simulink model "AcermanDynExt"  (R2019b)
settings: Solver=FixedStepAuto  StartTime=0.0  StopTime=simTime  RelTol=1e-3
values from neighbouring files (symbols this model uses):
  a0 = 1    [Ackerman_init.m]
  a1 = 4    [Ackerman_init.m]
  a2 = 3    [Ackerman_init.m]
  Change = 0    [Ackerman_init.m]
  k0 = 1    [Ackerman_init.m]
  k1 = place(Ad,bd,pd)    [Ackerman_init.m]
  k2 = place(Ac,bc,lambdatr')    [Ackerman_init.m]
  l = ylabel('$\omega(t)$' )    [Ackerman_init.m]
  pathType = 1    [Ackerman_init.m]
  phi0 = 0    [Ackerman_init.m]
  r = 2    [Ackerman_init.m]
  ref0 = [0 0]'    [Ackerman_init.m]
  refType = 1    [Ackerman_init.m]
  T = 0.324    [Ackerman_init.m]
  theta0 = pi/2    (= 1.57079632679)    [Ackerman_init.m]
  v0 = 1    [Ackerman_init.m]
  v_ref = 2    [Ackerman_init.m]
  x0 = 1    [Ackerman_init.m]
  y0 = 1    [Ackerman_init.m]
libraries: robotmobilelib x5
(part 1 of 6)
settings Model: Creator=mohd-  LastModifiedBy=mohd-

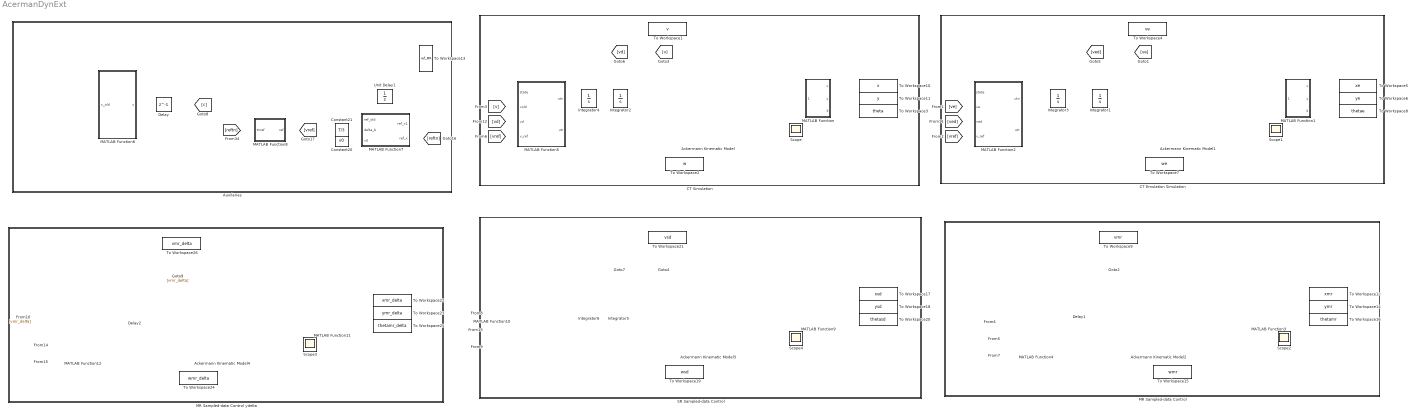
== system AcermanDynExt ==
  Ackermann Kinematic Model{,1..4} (5 alike) : robotmobilelib/Ackermann Kinematic Model  WheelBase=l  VehicleSpeedRange=[-inf inf]  MaxSteeringAngle=pi/3  InitialState=[x0; y0; theta0; phi0]  SimulateUsing=Interpreted execution
      settings: SourceProductName=Robotics System Toolbox  SourceProductBaseCode=RO
  Auxilaries : Subsystem
  CT Emulation Simulation : Subsystem
  CT Simulation : Subsystem
  Constant20 : Constant  Value=v0
  Constant21 : Constant  Value=T/3
  Delay : Delay  DelayLength=1  InitialCondition=0  SampleTime=T/3
  Delay1 : Delay  DelayLength=1  InitialCondition=v0  SampleTime=T
  Delay2 : Delay  DelayLength=1  InitialCondition=v0  SampleTime=T
  Integrator1 : Integrator  InitialCondition=v0
  Integrator2 : Integrator  InitialCondition=v0
  Integrator3 : Integrator
  Integrator4 : Integrator
  Integrator5 : Integrator  InitialCondition=v0
  Integrator6 : Integrator
  MATLAB Function : MATLAB Function  TreatAsAtomicUnit=on
  MATLAB Function1 : MATLAB Function  TreatAsAtomicUnit=on
  MATLAB Function10 : MATLAB Function  TreatAsAtomicUnit=on  SystemSampleTime=T
  MATLAB Function11 : MATLAB Function  TreatAsAtomicUnit=on
  MATLAB Function12 : MATLAB Function  TreatAsAtomicUnit=on  SystemSampleTime=T
  MATLAB Function2 : MATLAB Function  TreatAsAtomicUnit=on  SystemSampleTime=T
  MATLAB Function3 : MATLAB Function  TreatAsAtomicUnit=on
  MATLAB Function4 : MATLAB Function  TreatAsAtomicUnit=on  SystemSampleTime=T
  MATLAB Function5 : MATLAB Function  TreatAsAtomicUnit=on
  MATLAB Function6 : MATLAB Function  TreatAsAtomicUnit=on  SystemSampleTime=T/3
  MATLAB Function7 : MATLAB Function  TreatAsAtomicUnit=on  SystemSampleTime=T
  MATLAB Function8 : MATLAB Function  TreatAsAtomicUnit=on
  MATLAB Function9 : MATLAB Function  TreatAsAtomicUnit=on
  MR Sampled-data Control : Subsystem
  MR Sampled-data Control ydelta : Subsystem
  SR Sampled-data Control : Subsystem
  Scope{,1..4} (5 alike) : Scope
  To Workspace1 : ToWorkspace  VariableName=v  SampleTime=10^-3
      settings: Save2DSignal=2-D array (concatenate along first dimension)
  To Workspace10 : ToWorkspace  VariableName=x  SampleTime=10^-3
      settings: Save2DSignal=2-D array (concatenate along first dimension)
  To Workspace11 : ToWorkspace  VariableName=y  SampleTime=10^-3
      settings: Save2DSignal=2-D array (concatenate along first dimension)
  To Workspace12 : ToWorkspace  VariableName=xmr  SampleTime=10^-3
      settings: Save2DSignal=2-D array (concatenate along first dimension)
  To Workspace13 : ToWorkspace  VariableName=ref_MR  SampleTime=T/3
  To Workspace14 : ToWorkspace  VariableName=ymr  SampleTime=10^-3
      settings: Save2DSignal=2-D array (concatenate along first dimension)
  To Workspace15 : ToWorkspace  VariableName=wmr  SampleTime=10^-3
      settings: Save2DSignal=2-D array (concatenate along first dimension)
  To Workspace16 : ToWorkspace  VariableName=thetamr  SampleTime=10^-3
      settings: Save2DSignal=2-D array (concatenate along first dimension)
  To Workspace17 : ToWorkspace  VariableName=xsd  SampleTime=10^-3
      settings: Save2DSignal=2-D array (concatenate along first dimension)
  To Workspace18 : ToWorkspace  VariableName=ysd  SampleTime=10^-3
      settings: Save2DSignal=2-D array (concatenate along first dimension)
  To Workspace19 : ToWorkspace  VariableName=wsd  SampleTime=10^-3
      settings: Save2DSignal=2-D array (concatenate along first dimension)
  To Workspace2 : ToWorkspace  VariableName=w  SampleTime=10^-3
      settings: Save2DSignal=2-D array (concatenate along first dimension)
  To Workspace20 : ToWorkspace  VariableName=thetasd  SampleTime=10^-3
      settings: Save2DSignal=2-D array (concatenate along first dimension)
  To Workspace21 : ToWorkspace  VariableName=vsd  SampleTime=10^-3
      settings: Save2DSignal=2-D array (concatenate along first dimension)
  To Workspace22 : ToWorkspace  VariableName=xmr_delta  SampleTime=10^-3
      settings: Save2DSignal=2-D array (concatenate along first dimension)
  To Workspace23 : ToWorkspace  VariableName=ymr_delta  SampleTime=10^-3
      settings: Save2DSignal=2-D array (concatenate along first dimension)
  To Workspace24 : ToWorkspace  VariableName=wmr_delta  SampleTime=10^-3
      settings: Save2DSignal=2-D array (concatenate along first dimension)
  To Workspace25 : ToWorkspace  VariableName=thetamr_delta  SampleTime=10^-3
      settings: Save2DSignal=2-D array (concatenate along first dimension)
  To Workspace26 : ToWorkspace  VariableName=vmr_delta  SampleTime=10^-3
      settings: Save2DSignal=2-D array (concatenate along first dimension)
  To Workspace3 : ToWorkspace  VariableName=theta  SampleTime=10^-3
      settings: Save2DSignal=2-D array (concatenate along first dimension)
  To Workspace4 : ToWorkspace  VariableName=ve  SampleTime=10^-3
      settings: Save2DSignal=2-D array (concatenate along first dimension)
  To Workspace5 : ToWorkspace  VariableName=xe  SampleTime=10^-3
      settings: Save2DSignal=2-D array (concatenate along first dimension)
  To Workspace6 : ToWorkspace  VariableName=ye  SampleTime=10^-3
      settings: Save2DSignal=2-D array (concatenate along first dimension)
  To Workspace7 : ToWorkspace  VariableName=we  SampleTime=10^-3
      settings: Save2DSignal=2-D array (concatenate along first dimension)
  To Workspace8 : ToWorkspace  VariableName=thetae  SampleTime=10^-3
      settings: Save2DSignal=2-D array (concatenate along first dimension)
  To Workspace9 : ToWorkspace  VariableName=vmr  SampleTime=10^-3
      settings: Save2DSignal=2-D array (concatenate along first dimension)
  Unit Delay1 : UnitDelay  InitialCondition=ref0  SampleTime=T/3  HasFrameUpgradeWarning=on
  wires:
  Ackermann Kinematic Model3/2 -> Scope4/1
  Ackermann Kinematic Model2/1 -> MATLAB Function4/1(state), MATLAB Function3/1(state)
  [vmr] -> MATLAB Function4/2(v)
  Constant20/1 -> MATLAB Function7/3(v0)
  MATLAB Function9/2(y) -> To Workspace18/1
  Delay1/1 -> To Workspace9/1, [vmr], Ackermann Kinematic Model2/1
  MATLAB Function3/1(x) -> To Workspace12/1
  MATLAB Function3/2(y) -> To Workspace14/1
  Ackermann Kinematic Model2/2 -> Scope2/1
  Ackermann Kinematic Model/1 -> MATLAB Function5/1(state), MATLAB Function/1(state)
  MATLAB Function1/1(x) -> To Workspace5/1
  Delay/1 -> [c], MATLAB Function6/1(c_old)
  MATLAB Function9/1(x) -> To Workspace17/1
  MATLAB Function1/3(theta) -> To Workspace8/1
  MATLAB Function10/2(utr) -> To Workspace19/1, Ackermann Kinematic Model3/2
  MATLAB Function3/3(theta) -> To Workspace16/1
  MATLAB Function4/1(u) -> Delay1/1
  MATLAB Function5/1(utn) -> Integrator4/1
  [vref] -> MATLAB Function10/4(v_ref)
  MATLAB Function6/1(c) -> Delay/1
  [c] -> MATLAB Function4/4(c)
  MATLAB Function8/1(ref) -> [vref]
  [v] -> MATLAB Function5/2(vold)
  Ackermann Kinematic Model/2 -> Scope/1
  [vref] -> MATLAB Function5/4(v_ref)
  MATLAB Function2/1(utn) -> Integrator3/1
  Integrator2/1 -> To Workspace1/1, [v], Ackermann Kinematic Model/1
  MATLAB Function/1(x) -> To Workspace10/1
  MATLAB Function/3(theta) -> To Workspace3/1
  [ve] -> MATLAB Function2/2(ve)
  MATLAB Function/2(y) -> To Workspace11/1
  Ackermann Kinematic Model1/2 -> Scope1/1
  MATLAB Function2/2(utr) -> To Workspace7/1, Ackermann Kinematic Model1/2
  MATLAB Function9/3(theta) -> To Workspace20/1
  MATLAB Function7/1(ref_x1) -> To Workspace13/1, Unit Delay1/1
  [vref] -> MATLAB Function2/4(v_ref)
  Ackermann Kinematic Model1/1 -> MATLAB Function2/1(state), MATLAB Function1/1(state)
  Ackermann Kinematic Model3/1 -> MATLAB Function10/1(state), MATLAB Function9/1(state)
  MATLAB Function1/2(y) -> To Workspace6/1
  MATLAB Function5/2(utr) -> To Workspace2/1, Ackermann Kinematic Model/2
  [vsd] -> MATLAB Function10/2(v)
  MATLAB Function7/2(ref_x) -> [reftn]
  [vref] -> MATLAB Function4/3(v_ref)
  [reftn] -> MATLAB Function8/1(tnref)
  Integrator1/1 -> To Workspace4/1, [ve], Ackermann Kinematic Model1/1
  Constant21/1 -> MATLAB Function7/2(delta_b)
  MATLAB Function10/1(utn) -> Integrator6/1
  Integrator5/1 -> To Workspace21/1, [vsd], Ackermann Kinematic Model3/1
  MATLAB Function4/2(w) -> To Workspace15/1, Ackermann Kinematic Model2/2
  Unit Delay1/1 -> MATLAB Function7/1(ref_old)
  Integrator3/1 -> [ved], Integrator1/1
  [ved] -> MATLAB Function2/3(ved)
  Integrator4/1 -> [vd], Integrator2/1
  [vd] -> MATLAB Function5/3(vd)
  Integrator6/1 -> [vsdd], Integrator5/1
  [vsdd] -> MATLAB Function10/3(vsdd)
  MATLAB Function11/1(x) -> To Workspace22/1
  MATLAB Function12/2(w) -> To Workspace24/1, Ackermann Kinematic Model4/2
  MATLAB Function11/2(y) -> To Workspace23/1
  Ackermann Kinematic Model4/2 -> Scope3/1
  Delay2/1 -> To Workspace26/1, [vmr_delta], Ackermann Kinematic Model4/1
  [vref] -> MATLAB Function12/3(v_ref)
  MATLAB Function12/1(u) -> Delay2/1
  [c] -> MATLAB Function12/4(c)
  MATLAB Function11/3(theta) -> To Workspace25/1
  Ackermann Kinematic Model4/1 -> MATLAB Function12/1(state), MATLAB Function11/1(state)
  [vmr_delta] -> MATLAB Function12/2(v)

== system AcermanDynExt/Auxilaries ==

== system AcermanDynExt/CT Emulation Simulation ==

== system AcermanDynExt/CT Simulation ==

== system AcermanDynExt/MR Sampled-data Control ==

== system AcermanDynExt/MR Sampled-data Control ydelta ==

== system AcermanDynExt/SR Sampled-data Control ==

== matlab function AcermanDynExt/MATLAB Function ==
  data: x output; state input; y output; theta output
function [x, y, theta] = fcn(state)

x = state(1);
y = state(2);
theta = state(3);

== matlab function AcermanDynExt/MATLAB Function5 ==
  data: state input; vold input; vd input; v_ref input; pathType parameter; k0 parameter; r parameter; l parameter; utn output; utr output; Change parameter; k2 parameter
function [utn,utr] = MATLAB_Function5(state, vold, vd, v_ref, pathType, k0, r, l, Change, k2)

x = state(1); y = state(2); theta = state(3); phi = state(4);
eta1 = vold; eta2 = vd;

if pathType == 1
    D = [ -(y*cos(theta) - x*sin(theta))/(x^2 + y^2), (eta1^2*(x*cos(theta) + y*sin(theta)))/(l*cos(phi)^2*(x^2 + y^2));
            2*x*cos(theta) + 2*y*sin(theta),           (2*eta1^2*(y*cos(theta) - x*sin(theta)))/(l*cos(phi)^2)];
    F  = [  (eta1*(sin(phi)*x^2 - 2*l*cos(phi)*sin(theta)*x + sin(phi)*y^2 + 2*l*cos(phi)*cos(theta)*y)*(eta1^2*l*x^2*cos(phi) - 3*eta1^2*l*y^2*cos(phi) + eta1^2*y^3*cos(theta)*sin(phi) - eta1^2*x^3*sin(phi)*sin(theta) + eta1^2*x^2*y*cos(theta)*sin(phi) - eta1^2*x*y^2*sin(phi)*sin(theta) - 4*eta1^2*l*x^2*cos(phi)*cos(theta)^2 + 4*eta1^2*l*y^2*cos(phi)*cos(theta)^2 + 3*eta2*l*x^3*cos(phi)*cos(theta) + 3*eta2*l*y^3*cos(phi)*sin(theta) + 3*eta2*l*x*y^2*cos(phi)*cos(theta) + 3*eta2*l*x^2*y*cos(phi)*sin(theta) - 8*eta1^2*l*x*y*cos(phi)*cos(theta)*sin(theta)))/(l^2*cos(phi)^2*(x^2 + y^2)^3);
                                                                                                                                                                                                                                                                                                                                           (2*eta1*(3*eta2*l^2*cos(phi)^2*sin(theta)^2 - eta1^2*x*cos(theta)*sin(phi)^2 - eta1^2*y*sin(phi)^2*sin(theta) + 3*eta2*l^2*cos(phi)^2*cos(theta)^2 + 3*eta2*l*y*cos(phi)*cos(theta)*sin(phi) - 3*eta2*l*x*cos(phi)*sin(phi)*sin(theta)))/(l^2*cos(phi)^2)];
else

    D = [ -(y*cos(theta)-x*sin(theta))/(x^2 + y^2),  (eta1^2*(x*cos(theta)+y*sin(theta)))/(cos(phi)^2*(x^2+y^2));
         4*x*cos(theta)*(x^2 + y^2-9)+4*y*sin(theta)*(x^2 + y^2+9),    eta1*(tan(phi)^2+1)*(4*y*eta1*cos(theta)*(x^2 + y^2+9)-4*x*eta1*sin(theta)*(x^2 + y^2-9))];
 
     F  = [ (eta1*(sin(phi)*x^2-2*cos(phi)*sin(theta)*x+sin(phi)*y^2+2*cos(theta)*cos(phi)*y)*(x^2*eta1^2*cos(phi)-3*y^2*eta1^2*cos(phi)-4*x^2*eta1^2*cos(theta)^2*cos(phi)+4*y^2*eta1^2*cos(theta)^2*cos(phi)+3*x^3*eta2*cos(theta)*cos(phi)+3*y^3*eta2*cos(phi)*sin(theta)+y^3*eta1^2*cos(theta)*sin(phi)-x^3*eta1^2*sin(theta)*sin(phi)+x^2*y*eta1^2*cos(theta)*sin(phi)-x*y^2*eta1^2*sin(theta)*sin(phi)+3*x*y^2*eta2*cos(theta)*cos(phi)+3*x^2*y*eta2*cos(phi)*sin(theta)-8*x*y*eta1^2*cos(theta)*cos(phi)*sin(theta)))/(cos(phi)^2*(x^2 + y^2)^3);
       (36*x*eta1^3*cos(theta) + 108*eta1*eta2*cos(phi)^2 - 36*y*eta1^3*sin(theta) - 4*x^3*eta1^3*cos(theta) - 4*y^3*eta1^3*sin(theta) + 4*x^3*eta1^3*cos(theta)*cos(phi)^2 + 4*y^3*eta1^3*cos(phi)^2*sin(theta) - 4*x*y^2*eta1^3*cos(theta) + 12*x^2*eta1*eta2*cos(phi)^2 + 36*y^2*eta1*eta2*cos(phi)^2 - 12*x*y*eta1^3*sin(2*phi) - 4*x^2*y*eta1^3*sin(theta) - 12*x*eta1^3*cos(theta)*cos(phi)^2 - 216*eta1*eta2*cos(theta)^2*cos(phi)^2 + 60*y*eta1^3*cos(phi)^2*sin(theta) + 4*x*y^2*eta1^3*cos(theta)*cos(phi)^2 + 24*x^2*eta1*eta2*cos(theta)^2*cos(phi)^2 - 24*y^2*eta1*eta2*cos(theta)^2*cos(phi)^2 + 4*x^2*y*eta1^3*cos(phi)^2*sin(theta) + 216*eta1^3*cos(theta)*cos(phi)*sin(theta)*sin(phi) + 48*x*y*eta1^3*cos(theta)^2*cos(phi)*sin(phi) + 108*y*eta1*eta2*cos(theta)*cos(phi)*sin(phi) + 108*x*eta1*eta2*cos(phi)*sin(theta)*sin(phi) - 24*x^2*eta1^3*cos(theta)*cos(phi)*sin(theta)*sin(phi) + 24*y^2*eta1^3*cos(theta)*cos(phi)*sin(theta)*sin(phi) + 12*y^3*eta1*eta2*cos(theta)*cos(phi)*sin(phi) - 12*x^3*eta1*eta2*cos(phi)*sin(theta)*sin(phi) + 48*x*y*eta1*eta2*cos(theta)*cos(phi)^2*sin(theta) + 12*x^2*y*eta1*eta2*cos(theta)*cos(phi)*sin(phi) - 12*x*y^2*eta1*eta2*cos(phi)*sin(theta)*sin(phi))/cos(phi)^2];
    
end

  
Di = pinv(D);

if pathType == 1
    alpha = x^2+y^2 - r^2;
    psi1 = x^2+y^2-r^2; %
    psi2 = 2*eta1*(x*cos(theta) + y*sin(theta));
    psi3 = 2*eta1^2*cos(theta)^2 + 2*eta1^2*sin(theta)^2 + eta2*(2*x*cos(theta) + 2*y*sin(theta)) + (2*eta1^2*tan(phi)*(y*cos(theta) - x*sin(theta)))/l;

else
    a       = 3; b       = 1.05*a;
    alpha = (x^2+y^2+a^2)^2-4*a^2*x^2-b^4; % defines the path
    psi1 = (x^2+y^2+a^2)^2-4*a^2*x^2-b^4;
    psi2 = 4*x*eta1*cos(theta)*(x^2 + y^2 - 9) + 4*y*eta1*sin(theta)*(x^2 + y^2 + 9);
    psi3 = eta2*(4*x*cos(theta)*(x^2 + y^2 - 9) + 4*y*sin(theta)*(x^2 + y^2 + 9)) + eta1*cos(theta)*(8*x^2*eta1*cos(theta) + 4*eta1*cos(theta)*(x^2 + y^2 - 9) + 8*x*y*eta1*sin(theta)) + eta1*sin(theta)*(8*y^2*eta1*sin(theta) + 4*eta1*sin(theta)*(x^2 + y^2 + 9) + 8*x*y*eta1*cos(theta)) + eta1*tan(phi)*(4*y*eta1*cos(theta)*(x^2 + y^2 + 9) - 4*x*eta1*sin(theta)*(x^2 + y^2 - 9));
end

if alpha < 1e-2 && Change == 1
    ref = 2*v_ref;
else
    ref = v_ref;
end
v1 = -k0*(eta1-ref)-k0*eta2; 
v2 = k2*[psi1;psi2;psi3];

u  = Di*([v1;v2]-F);
utn = u(1); 
utr = u(2);

== matlab function AcermanDynExt/MATLAB Function1 ==
  data: x output; state input; y output; theta output
function [x, y, theta] = fcn(state)

x = state(1);
y = state(2);
theta = state(3);

== matlab function AcermanDynExt/MATLAB Function2 ==
  data: state input; ve input; ved input; v_ref input; pathType parameter; k0 parameter; r parameter; l parameter; utn output; utr output; Change parameter; k2 parameter
function [utn,utr] = MATLAB_Function2(state, ve, ved,v_ref, pathType, k0, r, l, Change, k2)

x = state(1); y = state(2); theta = state(3); phi = state(4);
eta1 = ve; eta2 = ved;


if pathType == 1
    D = [ -(y*cos(theta) - x*sin(theta))/(x^2 + y^2), (eta1^2*(x*cos(theta) + y*sin(theta)))/(l*cos(phi)^2*(x^2 + y^2));
            2*x*cos(theta) + 2*y*sin(theta),           (2*eta1^2*(y*cos(theta) - x*sin(theta)))/(l*cos(phi)^2)];
    F  = [  (eta1*(sin(phi)*x^2 - 2*l*cos(phi)*sin(theta)*x + sin(phi)*y^2 + 2*l*cos(phi)*cos(theta)*y)*(eta1^2*l*x^2*cos(phi) - 3*eta1^2*l*y^2*cos(phi) + eta1^2*y^3*cos(theta)*sin(phi) - eta1^2*x^3*sin(phi)*sin(theta) + eta1^2*x^2*y*cos(theta)*sin(phi) - eta1^2*x*y^2*sin(phi)*sin(theta) - 4*eta1^2*l*x^2*cos(phi)*cos(theta)^2 + 4*eta1^2*l*y^2*cos(phi)*cos(theta)^2 + 3*eta2*l*x^3*cos(phi)*cos(theta) + 3*eta2*l*y^3*cos(phi)*sin(theta) + 3*eta2*l*x*y^2*cos(phi)*cos(theta) + 3*eta2*l*x^2*y*cos(phi)*sin(theta) - 8*eta1^2*l*x*y*cos(phi)*cos(theta)*sin(theta)))/(l^2*cos(phi)^2*(x^2 + y^2)^3);
                                                                                                                                                                                                                                                                                                                                           (2*eta1*(3*eta2*l^2*cos(phi)^2*sin(theta)^2 - eta1^2*x*cos(theta)*sin(phi)^2 - eta1^2*y*sin(phi)^2*sin(theta) + 3*eta2*l^2*cos(phi)^2*cos(theta)^2 + 3*eta2*l*y*cos(phi)*cos(theta)*sin(phi) - 3*eta2*l*x*cos(phi)*sin(phi)*sin(theta)))/(l^2*cos(phi)^2)];
else

    D = [ -(y*cos(theta)-x*sin(theta))/(x^2 + y^2),  (eta1^2*(x*cos(theta)+y*sin(theta)))/(cos(phi)^2*(x^2+y^2));
         4*x*cos(theta)*(x^2 + y^2-9)+4*y*sin(theta)*(x^2 + y^2+9),    eta1*(tan(phi)^2+1)*(4*y*eta1*cos(theta)*(x^2 + y^2+9)-4*x*eta1*sin(theta)*(x^2 + y^2-9))];
 
     F  = [ (eta1*(sin(phi)*x^2-2*cos(phi)*sin(theta)*x+sin(phi)*y^2+2*cos(theta)*cos(phi)*y)*(x^2*eta1^2*cos(phi)-3*y^2*eta1^2*cos(phi)-4*x^2*eta1^2*cos(theta)^2*cos(phi)+4*y^2*eta1^2*cos(theta)^2*cos(phi)+3*x^3*eta2*cos(theta)*cos(phi)+3*y^3*eta2*cos(phi)*sin(theta)+y^3*eta1^2*cos(theta)*sin(phi)-x^3*eta1^2*sin(theta)*sin(phi)+x^2*y*eta1^2*cos(theta)*sin(phi)-x*y^2*eta1^2*sin(theta)*sin(phi)+3*x*y^2*eta2*cos(theta)*cos(phi)+3*x^2*y*eta2*cos(phi)*sin(theta)-8*x*y*eta1^2*cos(theta)*cos(phi)*sin(theta)))/(cos(phi)^2*(x^2 + y^2)^3);
       (36*x*eta1^3*cos(theta) + 108*eta1*eta2*cos(phi)^2 - 36*y*eta1^3*sin(theta) - 4*x^3*eta1^3*cos(theta) - 4*y^3*eta1^3*sin(theta) + 4*x^3*eta1^3*cos(theta)*cos(phi)^2 + 4*y^3*eta1^3*cos(phi)^2*sin(theta) - 4*x*y^2*eta1^3*cos(theta) + 12*x^2*eta1*eta2*cos(phi)^2 + 36*y^2*eta1*eta2*cos(phi)^2 - 12*x*y*eta1^3*sin(2*phi) - 4*x^2*y*eta1^3*sin(theta) - 12*x*eta1^3*cos(theta)*cos(phi)^2 - 216*eta1*eta2*cos(theta)^2*cos(phi)^2 + 60*y*eta1^3*cos(phi)^2*sin(theta) + 4*x*y^2*eta1^3*cos(theta)*cos(phi)^2 + 24*x^2*eta1*eta2*cos(theta)^2*cos(phi)^2 - 24*y^2*eta1*eta2*cos(theta)^2*cos(phi)^2 + 4*x^2*y*eta1^3*cos(phi)^2*sin(theta) + 216*eta1^3*cos(theta)*cos(phi)*sin(theta)*sin(phi) + 48*x*y*eta1^3*cos(theta)^2*cos(phi)*sin(phi) + 108*y*eta1*eta2*cos(theta)*cos(phi)*sin(phi) + 108*x*eta1*eta2*cos(phi)*sin(theta)*sin(phi) - 24*x^2*eta1^3*cos(theta)*cos(phi)*sin(theta)*sin(phi) + 24*y^2*eta1^3*cos(theta)*cos(phi)*sin(theta)*sin(phi) + 12*y^3*eta1*eta2*cos(theta)*cos(phi)*sin(phi) - 12*x^3*eta1*eta2*cos(phi)*sin(theta)*sin(phi) + 48*x*y*eta1*eta2*cos(theta)*cos(phi)^2*sin(theta) + 12*x^2*y*eta1*eta2*cos(theta)*cos(phi)*sin(phi) - 12*x*y^2*eta1*eta2*cos(phi)*sin(theta)*sin(phi))/cos(phi)^2];
    
end

  
Di = pinv(D);

if pathType == 1
    alpha = x^2+y^2 - r^2;
    psi1 = x^2+y^2-r^2; %
    psi2 = 2*eta1*(x*cos(theta) + y*sin(theta));
    psi3 = 2*eta1^2*cos(theta)^2 + 2*eta1^2*sin(theta)^2 + eta2*(2*x*cos(theta) + 2*y*sin(theta)) + (2*eta1^2*tan(phi)*(y*cos(theta) - x*sin(theta)))/l;

else
    a       = 3; b       = 1.05*a;
    alpha = (x^2+y^2+a^2)^2-4*a^2*x^2-b^4; % defines the path
    psi1 = (x^2+y^2+a^2)^2-4*a^2*x^2-b^4;
    psi2 = 4*x*eta1*cos(theta)*(x^2 + y^2 - 9) + 4*y*eta1*sin(theta)*(x^2 + y^2 + 9);
    psi3 = eta2*(4*x*cos(theta)*(x^2 + y^2 - 9) + 4*y*sin(theta)*(x^2 + y^2 + 9)) + eta1*cos(theta)*(8*x^2*eta1*cos(theta) + 4*eta1*cos(theta)*(x^2 + y^2 - 9) + 8*x*y*eta1*sin(theta)) + eta1*sin(theta)*(8*y^2*eta1*sin(theta) + 4*eta1*sin(theta)*(x^2 + y^2 + 9) + 8*x*y*eta1*cos(theta)) + eta1*tan(phi)*(4*y*eta1*cos(theta)*(x^2 + y^2 + 9) - 4*x*eta1*sin(theta)*(x^2 + y^2 - 9));
end

if alpha < 1e-2 && Change == 1
    ref = 2*v_ref;
else
    ref = v_ref;
end
v1 = -k0*(eta1-ref)-k0*eta2; 
v2 = k2*[psi1;psi2;psi3];

u  = Di*([v1;v2]-F);
utn = u(1); 
utr = u(2);

== matlab function AcermanDynExt/MATLAB Function3 ==
  data: x output; state input; y output; theta output
function [x, y, theta] = fcn(state)

x = state(1);
y = state(2);
theta = state(3);
